simulink model "BPSK_rc"  (R2022b)
settings: Solver=FixedStepDiscrete  StartTime=0.0  StopTime=tsim  FixedStep=1/100000  RelTol=1e-3  AbsTol=1e-6
values from neighbouring files (symbols this model uses):
  alfa = 0    [parte2.m]
  fc = 10e3    (= 10000)    [init_vars.m]
  rb = 1e3    (= 1000)    [init_vars.m]
undefined symbols (not defined in the file or in its folder): gcbh, rcfiltgaincompat
libraries: commrandsrc2 x1, commfilt2 x1
settings Model: Creator=bekom  LastModifiedBy=joaogaspar
settings SolverCC: AlgebraicLoopSolver=TrustRegion
settings DataIOCC: SaveFormat=Array  SignalLoggingSaveFormat=ModelDataLogs  ReturnWorkspaceOutputs=off
settings OptimizationCC: BlockReduction=off  BooleanDataType=off
settings DebuggingCC: SaveWithParameterizedLinksMsg=none  UnderspecifiedInitializationDetection=Classic  MergeDetectMultiDrivingBlocksExec=none  SignalResolutionControl=TryResolveAllWithWarning  MultiTaskDSMMsg=warning  MultiTaskCondExecSysMsg=none  UnconnectedInputMsg=warning  UnconnectedOutputMsg=warning  UnconnectedLineMsg=warning  SFMachineParentedDataDiag=warning
settings HardwareCC: TargetUnknown=on
settings ModelReferenceCC: EnableRefExpFcnMdlSchedulingChecks=on  PropagateSignalLabelsOutOfModel=off
settings SFSimCC: CustomCodeUndefinedFunction=UseInterfaceOnly
settings RTWCC: TemplateMakefile=grt_unix.tmf
settings GRTTargetCC: CombineOutputUpdateFcns=off  GRTInterface=on

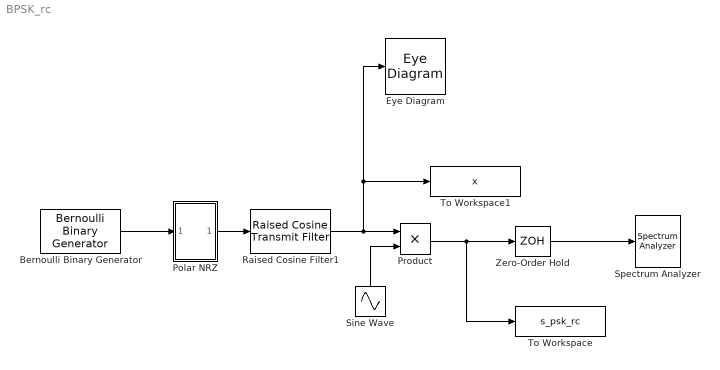
== system BPSK_rc ==
  Bernoulli Binary Generator : commrandsrc2/Bernoulli Binary Generator  P=0.5  seed=61  Ts=1/rb  frameBased=off  sampPerFrame=1  orient=off  outDataType=double
  Eye Diagram : EyeDiagram
  Polar NRZ : Subsystem  mask(Polar NRZ){}
      mask help:
      | This block encodes a unipolar NRZ signal into the polar NRZ line code
      |
      | The output values are +1 for a nonzero input and -1 for a zero one.
      mask Display: disp('Polar\nNRZ')
  Product : Product  InputSameDT=on  RndMeth=Zero  SaturateOnIntegerOverflow=on  OutDataTypeStr=Inherit: Same as first input
  Raised Cosine Filter1 : commfilt2/Raised Cosine Transmit Filter  filtType=Normal  R=alfa  filtSpan=10  N=100  filterGain=rcfiltgaincompat(gcbh)  InputProcessing=Columns as channels (frame based)  RateOptions=Allow multirate processing  framing=Mute  checkCoeff=off  variableName=rcTxFilt1  checkGain=Normalized  sampMode=Mute  saveAsFlag=0  currentFiltSpan=2*(5)  D=5  launchFVT=on  roundingMode=Floor  overflowMode=off  coeffDataTypeStr=Inherit: Same word length as input  coeffMin=[]  coeffMax=[]  coeffLastDataTypeStr=Inherit: Same word length as input  outputDataTypeStr=Inherit: Same as accumulator  outputMin=[]  outputMax=[]  outputLastDataTypeStr=Inherit: Same as accumulator
  Sine Wave : Sin  Frequency=2*pi*fc  SampleTime=0
  Spectrum Analyzer : SpectrumAnalyzer
  To Workspace : ToWorkspace  VariableName=s_psk_rc  SaveFormat=Timeseries  SampleTime=-1
  To Workspace1 : ToWorkspace  VariableName=x  SaveFormat=Timeseries  SampleTime=-1
  Zero-Order Hold : ZeroOrderHold  SampleTime=-1
  wires:
  Bernoulli Binary Generator/1 -> Polar NRZ/1(In1)
  Sine Wave/1 -> Product/2
  Product/1 -> To Workspace/1, Zero-Order Hold/1
  Zero-Order Hold/1 -> Spectrum Analyzer/1
  Raised Cosine Filter1/1 -> Eye Diagram/1, To Workspace1/1, Product/1
  Polar NRZ/1(Out1) -> Raised Cosine Filter1/1

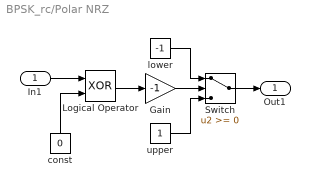
== system BPSK_rc/Polar NRZ ==
  In1 : Inport
  Gain : Gain  Gain=-1  SaturateOnIntegerOverflow=on  OutDataTypeStr=Inherit: Same as input  ParamDataTypeStr=Inherit: Same as input
  Logical Operator : Logic  Operator=XOR
  Switch : Switch
  const : Constant  Value=0
  lower : Constant  Value=-1
  upper : Constant
  Out1 : Outport  InitialOutput=0  VectorParamsAs1DForOutWhenUnconnected=off
  wires:
  const/1 -> Logical Operator/2
  Logical Operator/1 -> Gain/1
  Switch/1 -> Out1/1
  Gain/1 -> Switch/2
  upper/1 -> Switch/3
  lower/1 -> Switch/1
  In1/1 -> Logical Operator/1
